simulink model "Simulink_AM"  (R2021b)
settings: Solver=VariableStepAuto  StartTime=0.0  StopTime=10.0  RelTol=1e-3
model workspace (MAT data in the model file):
  fm = 2
  fp = 300
  fs = 5000
  m = 0.8
settings Model: Creator=enrique  LastModifiedBy=enrique
settings SolverCC: AlgebraicLoopSolver=TrustRegion
settings DebuggingCC: SFMachineParentedDataDiag=warning

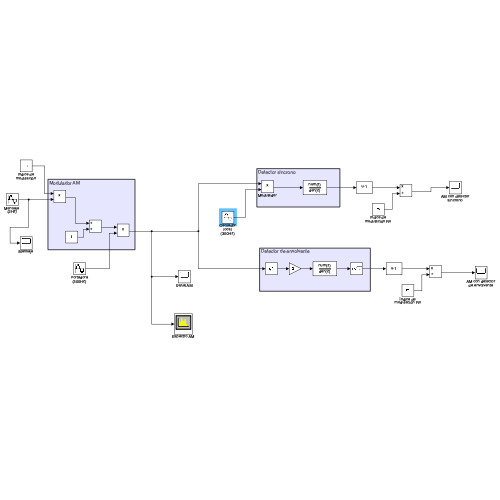
[thumbnail: Simulink's stored preview of the top-level diagram]
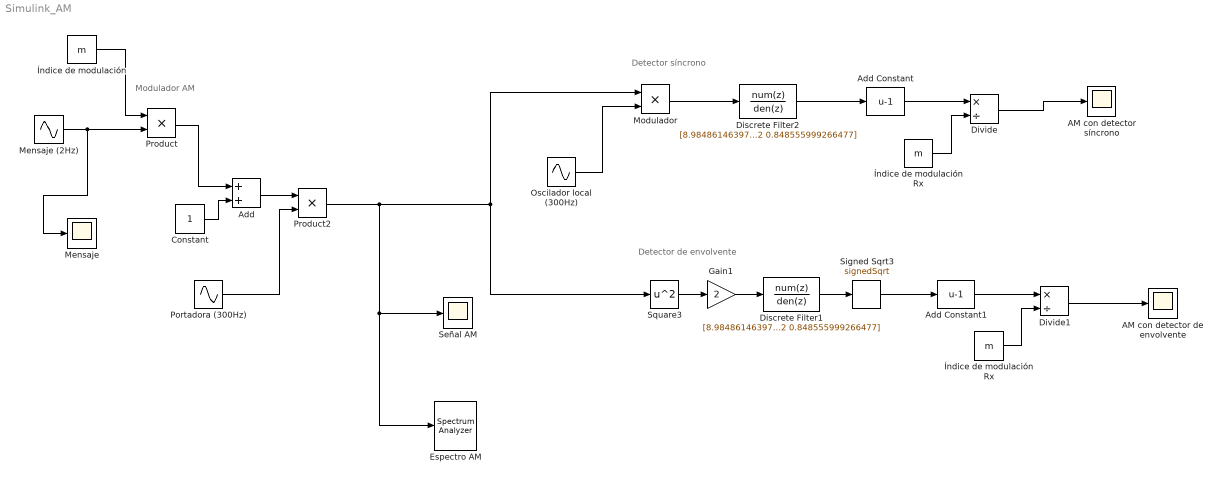
== system Simulink_AM ==
  note: Detector de envolvente
  note: Detector síncrono
  note: Modulador AM
  AM con detector de envolvente : Scope
  AM con detector síncrono : Scope
  Add : Sum
  Add Constant : Bias  Bias=-1
  Add Constant1 : Bias  Bias=-1
  Constant : Constant
  Discrete Filter1 : DiscreteFilter  Numerator="[8.98486146397045e-07\t3.59394458558818e-06\t5.39091687838227e-06\t3.59394458558818e-06\t8.98486146397045e-07]"  Denominator="[1\t-3.83582554064735\t5.52081913662223\t-3.53353521946302\t0.848555999266477]"  InputProcessing=Columns as channels (frame based)
  Discrete Filter2 : DiscreteFilter  Numerator="[8.98486146397045e-07\t3.59394458558818e-06\t5.39091687838227e-06\t3.59394458558818e-06\t8.98486146397045e-07]"  Denominator="[1\t-3.83582554064735\t5.52081913662223\t-3.53353521946302\t0.848555999266477]"  InputProcessing=Columns as channels (frame based)
  Divide : Product  Inputs=*/
  Divide1 : Product  Inputs=*/
  Espectro AM : SpectrumAnalyzer
  Gain1 : Gain  Gain=2
  Mensaje : Scope
  "Mensaje (2Hz) " : Sin  Frequency=2*pi*fm  SampleTime=1/fs
  Modulador : Product  OutDataTypeStr=Inherit: Same as first input
  Oscilador local (300Hz) : Sin  Amplitude=2  Frequency=2*pi*fp  SampleTime=1/fs
  "Portadora (300Hz) " : Sin  Frequency=2*pi*fp  SampleTime=1/fs
  Product : Product
  Product2 : Product  OutDataTypeStr=Inherit: Same as first input
  Señal AM : Scope
  Signed Sqrt3 : Sqrt  Operator=signedSqrt  SaturateOnIntegerOverflow=on
  Square3 : Math  Operator=square  SaturateOnIntegerOverflow=on
  Índice de modulación : Constant  Value=m
  Índice de modulación Rx : Constant  Value=m
  "Índice de modulación Rx " : Constant  Value=m
  wires:
  Índice de modulación/1 -> Product/1
  Constant/1 -> Add/2
  Add/1 -> Product2/1
  Product/1 -> Add/1
  "Portadora (300Hz) "/1 -> Product2/2
  "Mensaje (2Hz) "/1 -> Product/2, Mensaje/1
  Oscilador local (300Hz)/1 -> Modulador/2
  Modulador/1 -> Discrete Filter2/1
  Discrete Filter1/1 -> Signed Sqrt3/1
  Square3/1 -> Gain1/1
  Gain1/1 -> Discrete Filter1/1
  Product2/1 -> Square3/1, Modulador/1, Señal AM/1, Espectro AM/1
  Discrete Filter2/1 -> Add Constant/1
  Divide/1 -> AM con detector síncrono/1
  Add Constant/1 -> Divide/1
  Índice de modulación Rx/1 -> Divide/2
  Add Constant1/1 -> Divide1/1
  "Índice de modulación Rx "/1 -> Divide1/2
  Signed Sqrt3/1 -> Add Constant1/1
  Divide1/1 -> AM con detector de envolvente/1
